simulink model "prep_model"  (R2022a)
settings: Solver=VariableStepAuto  StartTime=0.0  StopTime=100  RelTol=1e-3
values from neighbouring files (symbols this model uses):
  A1 = double(subs(A))    [Prep.m]
  B1 = double(subs(B))    [Prep.m]
  F1 = - place(A1,B1,p)    [Prep.m]
settings Model: Creator=theod  LastModifiedBy=theod

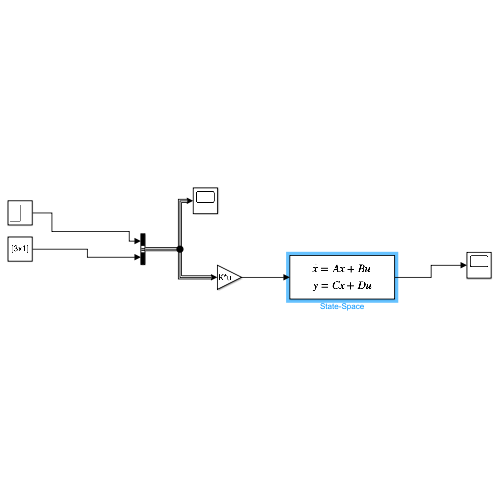
[thumbnail: Simulink's stored preview of the top-level diagram]
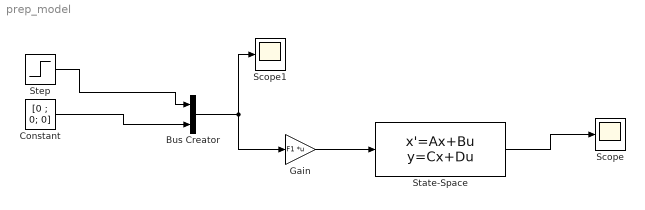
== system prep_model ==
  Bus Creator : BusCreator  Inputs=2
  Constant : Constant  Value=[0 ; 0; 0]
  Gain : Gain  Gain=F1  Multiplication=Matrix(K*u)
  Scope : Scope
  Scope1 : Scope
  State-Space : StateSpace  A=A1  B=B1  C=[1 0 0 0]  D=0  InitialCondition=0
  Step : Step  Time=0  SampleTime=0
  wires:
  State-Space/1 -> Scope/1
  Bus Creator/1 -> Scope1/1, Gain/1
  Step/1 -> Bus Creator/1
  Constant/1 -> Bus Creator/2
  Gain/1 -> State-Space/1
